simulink model "dc_simulink"  (R2024a)
settings: Solver=VariableStepAuto  StartTime=0.0  StopTime=10.0  RelTol=1e-3
values from neighbouring files (symbols this model uses):
  b = 0.0012    [DC.m]    (also in dc_parametros.m)
  J = 0.001    [DC.m]    (also in dc_parametros.m)
  Ke = 0.01    [DC.m]    (also in dc_parametros.m)
  Kt = Ke    (= 0.01)    [DC.m]    (also in dc_parametros.m)
  La = 0.023    [DC.m]    (also in dc_parametros.m)
  Ra = 2    [DC.m]    (also in dc_parametros.m)
settings Model: Creator=100117273  LastModifiedBy=100117273

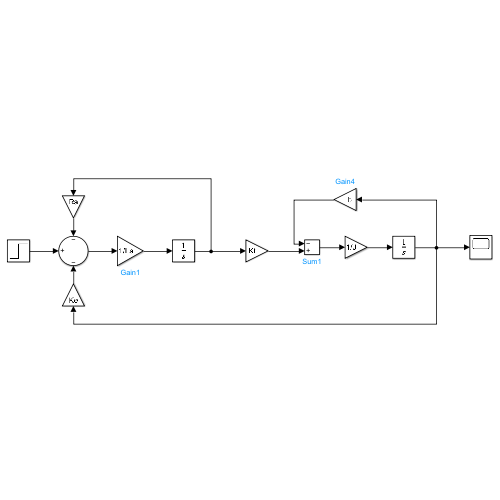
[thumbnail: Simulink's stored preview of the top-level diagram]
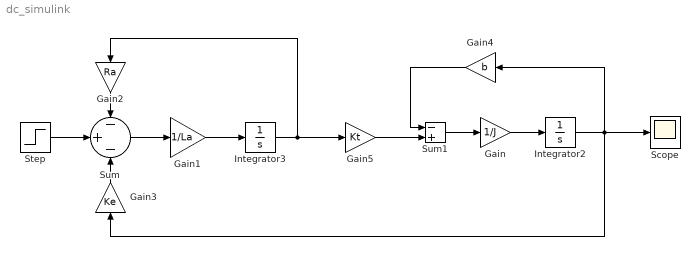
== system dc_simulink ==
  Gain : Gain  Gain=1/J
  Gain1 : Gain  Gain=1/La
  Gain2 : Gain  Gain=Ra
  Gain3 : Gain  Gain=Ke
  Gain4 : Gain  Gain=b
  Gain5 : Gain  Gain=Kt
  Integrator2 : Integrator
  Integrator3 : Integrator
  Scope : Scope
  Step : Step  Time=0  After=5  SampleTime=0
  Sum : Sum  Inputs=-+-
  Sum1 : Sum  Inputs=-+
  wires:
  Gain1/1 -> Integrator3/1
  Integrator3/1 -> Gain2/1, Gain5/1
  Gain/1 -> Integrator2/1
  Sum/1 -> Gain1/1
  Step/1 -> Sum/2
  Gain2/1 -> Sum/1
  Gain3/1 -> Sum/3
  Gain4/1 -> Sum1/1
  Gain5/1 -> Sum1/2
  Sum1/1 -> Gain/1
  Integrator2/1 -> Gain3/1, Scope/1, Gain4/1
